simulink model "gen_signal"  (R2021b)
settings: Solver=VariableStepAuto  StartTime=0.0  StopTime=1100  RelTol=1e-3
values from neighbouring files (symbols this model uses):
  SPEED_MAX = 3000    [gen_singal.m]
  Ts = 50e-3    (= 0.05)    [gen_singal.m]
settings Model: Creator=adria  LastModifiedBy=adria

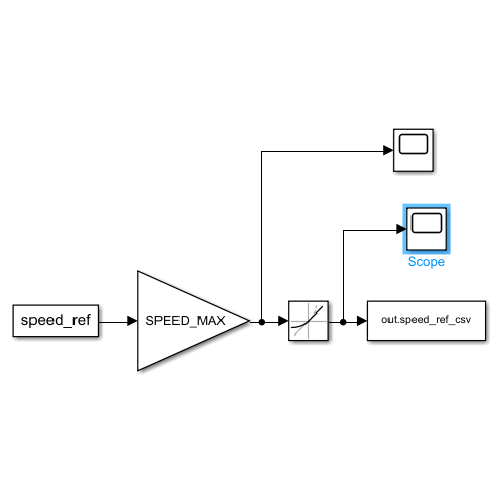
[thumbnail: Simulink's stored preview of the top-level diagram]
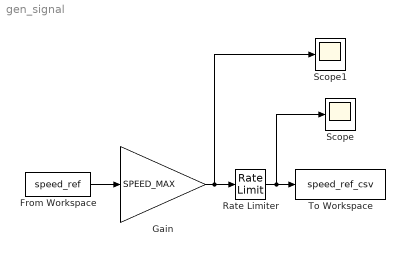
== system gen_signal ==
  From Workspace : FromWorkspace  VariableName=speed_ref  SampleTime=Ts
  Gain : Gain  Gain=SPEED_MAX
  Rate Limiter : RateLimiter  RisingSlewLimit=SPEED_MAX / 5  FallingSlewLimit=- SPEED_MAX / 5  SampleTimeMode=inherited
  Scope : Scope
  Scope1 : Scope
  To Workspace : ToWorkspace  VariableName=speed_ref_csv  SaveFormat=Timeseries  SampleTime=-1
  wires:
  From Workspace/1 -> Gain/1
  Gain/1 -> Scope1/1, Rate Limiter/1
  Rate Limiter/1 -> Scope/1, To Workspace/1
